simulink model "constantTorqueDemoReal"  (Simulink 7.6)
settings: Solver=ode45  StartTime=0.0  StopTime=inf  RelTol=1e-3
undefined symbols (not defined in the file or in its folder): PendulumVisualizer
libraries: robotlib x3, simulink x1
settings Model: Creator=russt  LastModifiedBy=russt

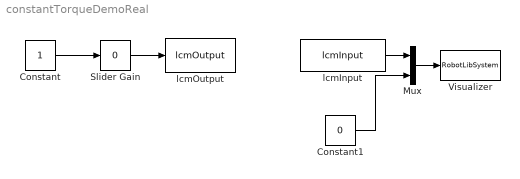
== system constantTorqueDemoReal ==
  Constant : Constant
  Constant1 : Constant  Value=0
  Mux : Mux  Inputs=2
  Slider Gain : simulink/Math Operations/Slider Gain  SystemSampleTime=-1  low=-5  gain=0  high=5
  Visualizer : robotlib/RobotLibSystem  sysobj=PendulumVisualizer()
  lcmInput : robotlib/lcmInput  channel='pendulum_y'  dim=1  decode_fcn=@(msg)decodeMeasurement(PendulumLCMCoder(),msg)  sample_time=.01
  lcmOutput : robotlib/lcmOutput  channel='pendulum_u'  dim=1  encode_fcn=@(t,u)encodeU(PendulumLCMCoder(),t,u)  sample_time=.01
  wires:
  Slider Gain/1 -> lcmOutput/1
  Constant/1 -> Slider Gain/1
  lcmInput/1 -> Mux/1
  Constant1/1 -> Mux/2
  Mux/1 -> Visualizer/1
